simulink model "quiz3"  (R2023b)
settings: Solver=VariableStepAuto  StartTime=0.0  StopTime=1  RelTol=1e-3

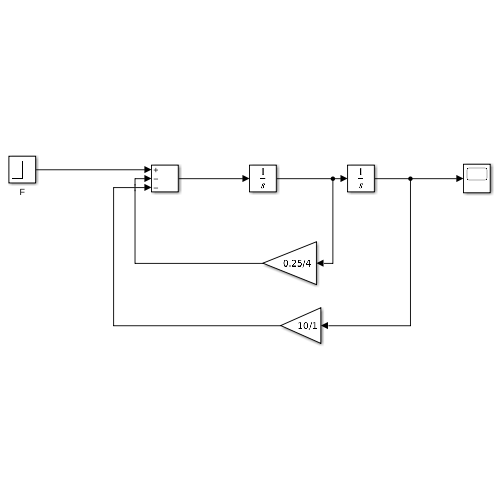
[thumbnail: Simulink's stored preview of the top-level diagram]
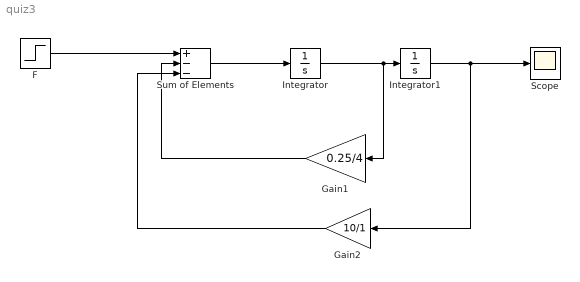
== system quiz3 ==
  F : Step  Time=2  After=100  SampleTime=0
  Gain1 : Gain  Gain=0.25/4
  Gain2 : Gain  Gain=10/1
  Integrator : Integrator
  Integrator1 : Integrator
  Scope : Scope
  Sum of Elements : Sum  Inputs=+--
  wires:
  Integrator/1 -> Gain1/1, Integrator1/1
  Integrator1/1 -> Gain2/1, Scope/1
  Sum of Elements/1 -> Integrator/1
  Gain1/1 -> Sum of Elements/2
  Gain2/1 -> Sum of Elements/3
  F/1 -> Sum of Elements/1
